simulink model "sgMdl_SCPI_PSU_Serial"  (R2024b)
settings: Solver=FixedStepAuto  StartTime=0.0  StopTime=inf  RelTol=1e-3
model workspace (MAT data in the model file):
  La_ratio = 0.5
libraries: speedgoatlib_serial_onboard x3, speedgoatlib_scpi x1
Description:
  | SCPI - PSU
settings Model: ModifiedByFormat=Speedgoat  SimulationMode=external  ExtModeEnableFloating=off  Creator=Speedgoat  LastModifiedBy=Speedgoat
settings SolverCC: ConcurrentTasks=on  PositivePriorityOrder=on
settings OptimizationCC: BlockReduction=off  OptimizeBlockIOStorage=off
settings DebuggingCC: UnderspecifiedInitializationDetection=Classic  MergeDetectMultiDrivingBlocksExec=none  TasksWithSamePriorityMsg=none
settings HardwareCC: ProdBitPerLong=64  ProdLongLongMode=on  ProdHWDeviceType=Intel->x86-64 (Linux 64)
settings ModelReferenceCC: PropagateSignalLabelsOutOfModel=off
settings RTWCC: Description=Speedgoat Real-Time Target Machine  SystemTargetFile=speedgoat.tlc  TemplateMakefile=slrealtime_default_tmf  Toolchain=Simulink Real-Time Toolchain  BuildConfiguration=Faster Runs  TargetLang=C++
settings SimulinkRealTimeTargetCC: SubcomponentCodeInterfacePackaging=Reusable function  InstructionSetFMA=off  LogToMDFFile=off  SLRTLogLevel=debug  SLRTFileLogMaxRuns=10
settings ConfigComp: CovBoundaryAbsTol=1.0e-5

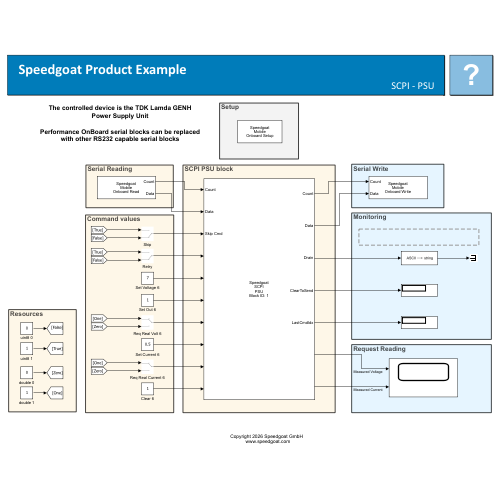
[thumbnail: Simulink's stored preview of the top-level diagram]
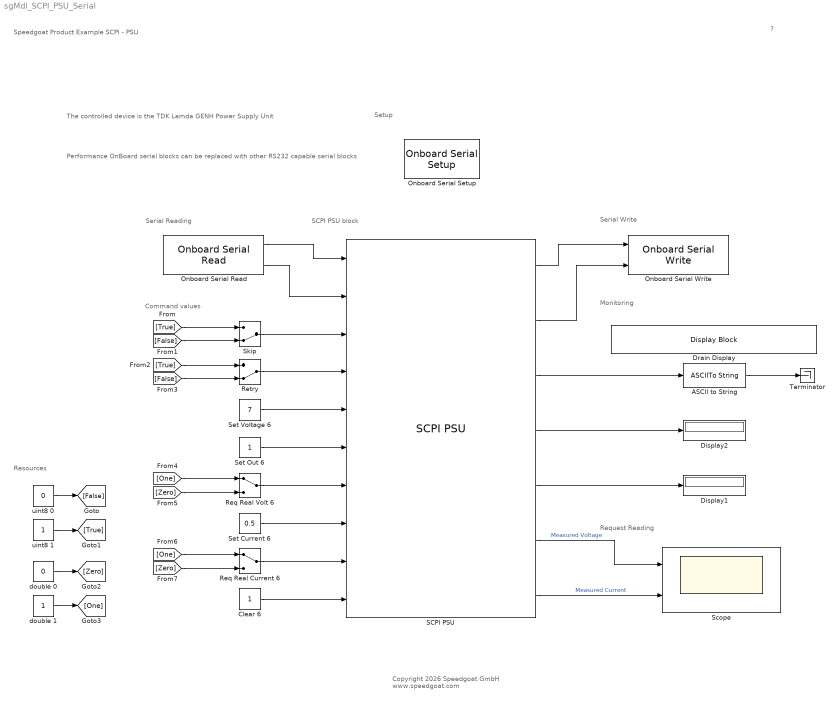
== system sgMdl_SCPI_PSU_Serial ==
  note: The controlled device is the TDK Lamda GENH Power Supply Unit
  note: Serial Reading
  note: Serial Write
  note: Setup
  note: Resources
  note: Monitoring
  note: Request Reading
  note: SCPI PSU block
  note: Performance OnBoard serial blocks can be replaced with other RS232 capable serial blocks
  note: Command values
  note: Speedgoat Product Example
      | SCPI - PSU
  note: ?
  note: Copyright 2026 Speedgoat GmbH
      |  www.speedgoat.com
  ASCII to String : ASCIIToString
  Clear 6 : Constant  OutDataTypeStr=double
  Display1 : Display
  Display2 : Display
  Drain Display : DisplayBlock  LabelPosition=Hide  Transparency=1
  Onboard Serial Read : speedgoatlib_serial_onboard/Onboard Serial Read  parMachineType=Performance  parPort=1  parSampleTime=-1  parEnLegacy=off  parDataType=8 bit uint null terminated  parRxSwFifoSize=64
      settings: SourceProductName=Onboard
  Onboard Serial Setup : speedgoatlib_serial_onboard/Onboard Serial Setup  parMachineType=Performance  parPort1=RS232  parPort2=Disabled  parPort3=Disabled  parPort4=Disabled  parEnCustBaud1=off  parCustBaudValue1=9600  parBaud1=9600  parParity1=None  parDataBits1=8  parStopBits1=1  parTxSwFifoSize1=64  parRxSwFifoSize1=64  parCtsMode1=off  parTerm1=on  parEnCustBaud2=off  parCustBaudValue2=9600  parBaud2=115200  parParity2=None  parDataBits2=8  parStopBits2=1  parTxSwFifoSize2=64  parRxSwFifoSize2=64  parCtsMode2=off  parTerm2=on  parEnCustBaud3=on  parCustBaudValue3=9600  parBaud3=115200  parParity3=None  parDataBits3=8  parStopBits3=1  parTxSwFifoSize3=64  parRxSwFifoSize3=64  parCtsMode3=on  parTerm3=on  parEnCustBaud4=on  parCustBaudValue4=9600  parBaud4=115200  parParity4=None  parDataBits4=8  parStopBits4=1  parTxSwFifoSize4=64  parRxSwFifoSize4=64  parCtsMode4=on  parTerm4=on
      settings: SourceProductName=Onboard
  Onboard Serial Write : speedgoatlib_serial_onboard/Onboard Serial Write  parMachineType=Performance  parPort=1  parSampleTime=-1  parEnLegacy=off  parDataType=8 bit uint null terminated  parMdlStopMsgEnable=on  parMdlStopMsgData="[\"GRST\"+char(13)]"  parMdlStopFifoOptions=Wait for the TX FIFO to empty  parMdlStopMsgsDataArr=[71 82 83 84 13]  parMdlStopMsgsDataSize=5  parTxSwFifoSize=64
      settings: SourceProductName=Onboard
  Req Real Current 6 : ManualSwitch
  Req Real Volt 6 : ManualSwitch
  Retry : ManualSwitch  CurrentSetting=0
  "SCPI PSU " : speedgoatlib_scpi/SCPI PSU   parDeviceInfo="compose([\"TDK Lambda\" \"GEN\" \"1\" \"Serial\" \"200000\" \"13\" \"13\" \"false\" \"['GRST' char(13)]\" \"true\" \"ADR <adr>\" \"OK\" \"true\" \"...\" \"Voltage\" \"Current\" \"Out State\" \"Foldback Protection\" \"Fold Back Delay\" \"OVP\" \"UVL\" \"Reset\" \"Clear Status\" \"...\" \"Volt\" \"Curr\" \"OutS\" \"FLD Prot\" \"FBD Delay\" \"OVP\" \"UVL\" \"RST\" \"CLS\" \"...\\n\" \"PV <value>\\n\" \"PC <value>\\n\" \"OUT <value>\\n\" \"FLD <value>\\n\" \"FBD <value>\\n\" \"OVP <value>\\n\" \"UVL <value>\\n\" \"RST\\n\" \"CLS\\n\" \"...\\n\" \"double\\n\" \"double\\n\" \"uint\\n\" \"double\\n\" \"double\\n\" \"double\\n\" \"double\\n\" \"none\\n\" \"none\\n\" \"...\\n\" \"OK\\n\" \"OK\\n\" \"OK\\n\" \"OK\\n\" \"OK\\n\" \"OK\\n\" \"OK\\n\" \"OK\\n\" \"OK\\n\" \"...\\n\" \"string\\n\" \"string\\n\" \"string\\n\" \"string\\n\" \"string\\n\" \"string\\n\" \"string\\n\" \"string\\n\" \"string\\n\" \"...\" \"Set Voltage\" \"Actual Voltage\" \"Set Current\" \"Actual Current\" \"Out State\" \"Foldback Protection\" \"Fold Back Delay\" \"OVP\" \"UVL\" \"...\" \"SetVolt\" \"RealV\" \"SetCurr\" \"RealCurr\" \"OutS\" \"FLD Prot\" \"FBD Delay\" \"OVP\" \"UVL\" \"...\\n\" \"PV?\\n\" \"MV?\\n\" \"PC?\\n\" \"MC?\\n\" \"OUT?\\n\" \"FLD?\\n\" \"FBD?\\n\" \"OVP?\\n\" \"UVL?\\n\" \"...\\n\" \"<value>\\n\" \"<value>\\n\" \"<value>\\n\" \"<value>\\n\" \"<value>\\n\" \"<value>\\n\" \"<value>\\n\" \"<value>\\n\" \"<value>\\n\" \"...\\n\" \"double\\n\" \"double\\n\" \"double\\n\" \"double\\n\" \"ON/OFF\\n\" \"double\\n\" \"double\\n\" \"double\\n\" \"double\\n\"])"  parId=1  parDeviceType=TDK Lambda GEN  parCommType=Serial  parTxFifoSize=64  parRxFifoSize=64  parSampleTime=-1  parInOutPortText=port_label('input', 5, '1#S6[Volt]');port_label('input', 6, '2#S6[OutS]');port_label('input', 7, '3#R6[RealV]');port_label('output', 6, '3#R6[RealV]');port_label('input', 8, '4#S6[Curr]');port_label('input', 9, '5#R6[RealCurr]');port_label('output', 7, '5#R6[RealCurr]');port_label('input', 10, '6#S6[CLS]');  parNCmds=6  parNReq=2  parCmdTypeArray=[1 1 2 1 2 1]  parMsgArray=[2 4 3 3 5 10]  parAddrArray=[6 6 6 6 6 6]  parChArray=[1 1 1 1 1 1]  parTableState=✅Command Table up to date  parEnTableNum=off  parCommandTable={ '6', '1', 'Voltage', '...'; '6', '1', 'Out State', '...'; '6', '1', '...', 'Actual Voltage'; '6', '1', 'Current', '...'; '6', '1', '...', 'Actual Current'; '6', '1', 'Clear Status', '...' }  parMdlStartMsgEnable=on  parMdlStartMsgData="{[\"GRST\"+char(13)]}"  parMdlStartMsgDelay=300  parMdlStartMsgsDataArr=[71 82 83 84 13]  parMdlStartMsgsSize=5  parShowCmdName=on  parShowAddr=on  parShowCh=on  parShowSkipCmd=on  parShowRetryCmd=on
      settings: SourceProductName=SCPI
  Scope : Scope  NumInputPorts=2
  Set Current 6 : Constant  Value=0.5  OutDataTypeStr=double
  Set Out 6 : Constant  OutDataTypeStr=double
  Set Voltage 6 : Constant  Value=7  OutDataTypeStr=double
  Skip : ManualSwitch  CurrentSetting=0
  Terminator : Terminator
  double 0 : Constant  Value=0  OutDataTypeStr=double
  double 1 : Constant  OutDataTypeStr=double
  uint8 0 : Constant  Value=0  OutDataTypeStr=uint8
  uint8 1 : Constant  OutDataTypeStr=uint8
  wires:
  Onboard Serial Read/1 -> "SCPI PSU "/1
  Onboard Serial Read/2 -> "SCPI PSU "/2
  uint8 0/1 -> [False]
  uint8 1/1 -> [True]
  [True] -> Skip/1
  [False] -> Skip/2
  [True] -> Retry/1
  [False] -> Retry/2
  [Zero] -> Req Real Volt 6/2
  [One] -> Req Real Volt 6/1
  [Zero] -> Req Real Current 6/2
  [One] -> Req Real Current 6/1
  double 0/1 -> [Zero]
  double 1/1 -> [One]
  Clear 6/1 -> "SCPI PSU "/10
  ASCII to String/1 -> Terminator/1
  Skip/1 -> "SCPI PSU "/3
  Retry/1 -> "SCPI PSU "/4
  Set Voltage 6/1 -> "SCPI PSU "/5
  Set Out 6/1 -> "SCPI PSU "/6
  Req Real Volt 6/1 -> "SCPI PSU "/7
  Set Current 6/1 -> "SCPI PSU "/8
  Req Real Current 6/1 -> "SCPI PSU "/9
  "SCPI PSU "/1 -> Onboard Serial Write/1
  "SCPI PSU "/2 -> Onboard Serial Write/2
  "SCPI PSU "/3 -> ASCII to String/1
  "SCPI PSU "/4 -> Display2/1
  "SCPI PSU "/5 -> Display1/1
  "SCPI PSU "/6 -> Scope/1  "Measured Voltage"
  "SCPI PSU "/7 -> Scope/2  "Measured Current"
